simulink model "STEVE_ver28"  (R2022a)
settings: Solver=VariableStepAuto  StartTime=0.0  StopTime=Stop_Time  FixedStep=0.000001  RelTol=1e-5
values from neighbouring files (symbols this model uses):
  Bed_ave_OD = (1+Bed_ins_OD)/2    (= 1.667)    [STEVE_initialization.m]    (also in STEVE_running.m = (1+Bed_ins_OD)/2; STEVE_v4_C1Demo_2023_Nominal.m)
  Bed_ins_OD = 2.334    [STEVE_initialization.m]    (also in STEVE_v4_C1Demo_2023_Nominal.m)
  Bed_thickness = 0.049    [STEVE_initialization.m]    (also in STEVE_v4_C1Demo_2023_Nominal.m)
  Belimo_Cv = 16    [STEVE_initialization.m]    (also in STEVE_v4_C1Demo_2023_Nominal.m)
  flow_rate = 8    [STEVE_initialization.m]    (also in STEVE_v4_C1Demo_2023_Nominal.m)
  Heat_ads = 40000    [STEVE_initialization.m]    (also in STEVE_v4_C1Demo_2023_Nominal.m)
  Heater_output = 85.3    [STEVE_initialization.m]    (also in STEVE_v4_C1Demo_2023_Nominal.m)
  L = 0.508    [STEVE_initialization.m]    (also in STEVE_v4_C1Demo_2023_Nominal.m)
  L_inch = L*39.3701    (= 20.0000108)    [STEVE_initialization.m]    (also in STEVE_v4_C1Demo_2023_Nominal.m)
  max_temp = 200+273.15    (= 473.15)    [STEVE_initialization.m]    (also in STEVE_v4_C1Demo_2023_Nominal.m)
  mesh_size = 15    [STEVE_initialization.m]    (also in STEVE_v4_C1Demo_2023_Nominal.m)
  Pipe_ave_HD = (pipe_HD+0.5)/2    (= 0.465)    [STEVE_initialization.m]    (also in STEVE_running.m = (pipe_HD+0.5)/2; STEVE_v4_C1Demo_2023_Nominal.m)
  pipe_HD = 0.43    [STEVE_initialization.m]    (also in STEVE_v4_C1Demo_2023_Nominal.m)
  Ramp_rate = 0.0833    [STEVE_initialization.m]    (also in STEVE_v4_C1Demo_2023_Nominal.m)
  room_pressure = 13.3    [STEVE_initialization.m]    (also in STEVE_v4_C1Demo_2023_Nominal.m)
  t_Total = Adsorption_time + FlowStop_time + Valve_close_Time + Select_valve_close_Time + Pump_down_time + Desorption_time + SelectValve_open_Time + Valve_open_Time    (= 9635)    [STEVE_initialization.m]    (also in STEVE_running.m = Adsorption_time + FlowStop_time + Valve_close_Time + Select_; STEVE_v4_C1Demo_2023_Nominal.m)
libraries: fl_lib x229, nesl_utility x75, slpidlib x2
(part 4 of 5)

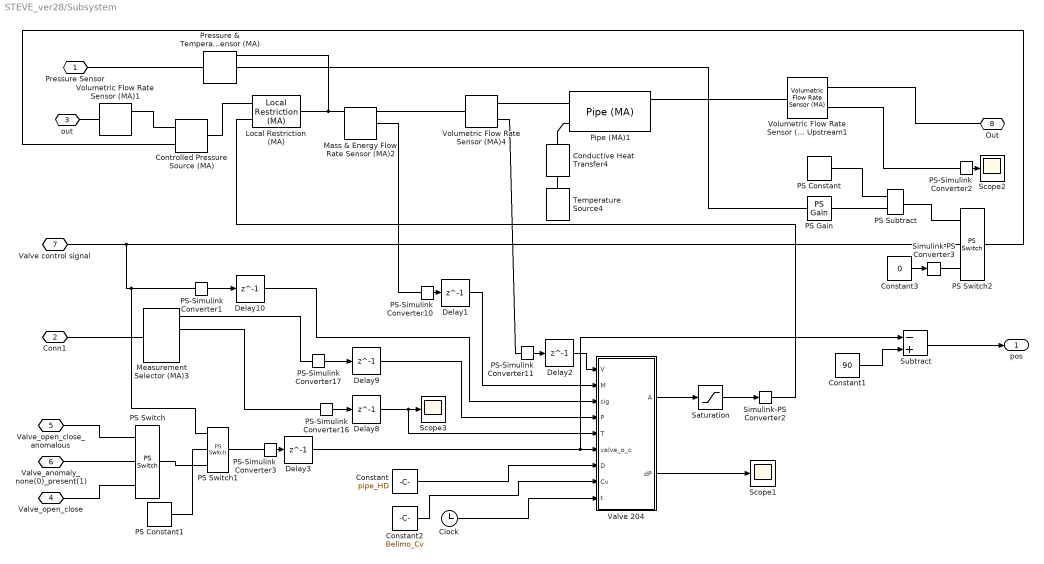
== system STEVE_ver28/Subsystem ==
  Clock : Clock
  Conductive Heat Transfer4 : fl_lib/Thermal/Thermal Elements/Conductive Heat Transfer  area=51.8 in^2  thickness=pipe_wall in  th_cond=pipe_tc W/(m*K)  T_specify=off  T_priority=None  T=0 K  T_nominal_specify=off  T_nominal_unit=K  T_nominal_value=1  Q_specify=off  Q_priority=None  Q=0 W  Q_nominal_specify=off  Q_nominal_unit=W  Q_nominal_value=1
      settings: SourceProductBaseCode=PW,SS,VE
  Constant : Constant  Value=pipe_HD
  Constant1 : Constant  Value=90
  Constant2 : Constant  Value=Belimo_Cv
  Constant3 : Constant  Value=0
  Controlled Pressure Source (MA) : fl_lib/Moist Air/Sources/Controlled Pressure Source (MA)  power_spec=foundation.enum.power_spec.isentropic  area_A=(pi*pipe_HD^2)/4 in^2  area_B=(pi*pipe_HD^2)/4 in^2
      settings: SourceProductBaseCode=PW,SS,VE  InternalSimscapePortConfiguration="{\"Bottom\":[],\"Left\":[{\"id\":\"A\",\"label\":\"A\",\"type\":\"foundation.moist_air.moist_air\"},{\"id\":\"P\",\"label\":\"P\",\"type\":\"input\"}],\"Right\":[{\"id\":\"B\",\"label\":\"B\",\"type\":\"foundation.moist_air.moist_air\"}],\"Top\":[]}"
  Delay1 : Delay  DelayLength=1  InitialCondition=0
  Delay10 : Delay  DelayLength=1  InitialCondition=0
  Delay2 : Delay  DelayLength=1  InitialCondition=0.00013
  Delay3 : Delay  DelayLength=1  InitialCondition=18
  Delay8 : Delay  DelayLength=1  InitialCondition=293
  Delay9 : Delay  DelayLength=1  InitialCondition=90000
  Local Restriction (MA) : fl_lib/Moist Air/Elements/Local Restriction (MA)  restriction_type=foundation.enum.restriction_type.variable  restriction_area=0.001 m^2  min_area=1e-20 in^2  max_area=(pi*(pipe_HD-0.0001)^2)/4 in^2  area=(pi*pipe_HD^2)/4 in^2  Cd=0.64  B_lam=0.999
      settings: SourceProductBaseCode=PW,SS,VE
  Mass & Energy Flow Rate Sensor (MA)2 : fl_lib/Moist Air/Sensors/Mass & Energy Flow Rate Sensor (MA)
      settings: SourceProductBaseCode=PW,SS,VE  InternalSimscapePortConfiguration="{\"Bottom\":[],\"Left\":[{\"id\":\"A\",\"label\":\"A\",\"type\":\"foundation.moist_air.moist_air\"},{\"id\":\"Mw\",\"label\":\"Mw\",\"type\":\"output\"},{\"id\":\"Mg\",\"label\":\"Mg\",\"type\":\"output\"}],\"Right\":[{\"id\":\"B\",\"label\":\"B\",\"type\":\"foundation.moist_air.moist_air\"},{\"id\":\"M\",\"label\":\"M\",\"type\":\"output\"},{\"id\":\"PHI\",\"label\":\"Phi\",\"type\":\"output\"}],\"Top\":[]}"
  Measurement Selector (MA)3 : fl_lib/Moist Air/Sensors/Measurement Selector (MA)  moisture_spec=foundation.enum.moisture_spec.relative_humidity  trace_gas_spec=foundation.enum.trace_gas_spec.mole_fraction
      settings: SourceProductBaseCode=PW,SS,VE
  PS Constant : fl_lib/Physical Signals/Sources/PS Constant  constant=0 Pa
      settings: SourceProductBaseCode=PW,SS,VE
  PS Constant1 : fl_lib/Physical Signals/Sources/PS Constant  constant=0
      settings: SourceProductBaseCode=PW,SS,VE
  PS Gain : fl_lib/Physical Signals/Functions/PS Gain  gain=1
      settings: SourceProductBaseCode=PW,SS,VE
  PS Subtract : fl_lib/Physical Signals/Functions/PS Subtract
      settings: SourceProductBaseCode=PW,SS,VE
  PS Switch : fl_lib/Physical Signals/Nonlinear Operators/PS Switch  Threshold=1
      settings: SourceProductBaseCode=PW,SS,VE  InternalSimscapePortConfiguration="{\"Bottom\":[],\"Left\":[{\"id\":\"I1\",\"label\":\"\",\"type\":\"input\"},{\"id\":\"I2\",\"label\":\"\",\"type\":\"input\"},{\"id\":\"I3\",\"label\":\"\",\"type\":\"input\"}],\"Right\":[{\"id\":\"O\",\"label\":\"\",\"type\":\"output\"}],\"Top\":[]}"
  PS Switch1 : fl_lib/Physical Signals/Nonlinear Operators/PS Switch  Threshold=1
      settings: SourceProductBaseCode=PW,SS,VE  InternalSimscapePortConfiguration="{\"Bottom\":[],\"Left\":[{\"id\":\"I1\",\"label\":\"\",\"type\":\"input\"},{\"id\":\"I2\",\"label\":\"\",\"type\":\"input\"},{\"id\":\"I3\",\"label\":\"\",\"type\":\"input\"}],\"Right\":[{\"id\":\"O\",\"label\":\"\",\"type\":\"output\"}],\"Top\":[]}"
  PS Switch2 : fl_lib/Physical Signals/Nonlinear Operators/PS Switch  Threshold=1
      settings: SourceProductBaseCode=PW,SS,VE  InternalSimscapePortConfiguration="{\"Bottom\":[],\"Left\":[{\"id\":\"I1\",\"label\":\"\",\"type\":\"input\"},{\"id\":\"I2\",\"label\":\"\",\"type\":\"input\"},{\"id\":\"I3\",\"label\":\"\",\"type\":\"input\"}],\"Right\":[{\"id\":\"O\",\"label\":\"\",\"type\":\"output\"}],\"Top\":[]}"
  PS-Simulink Converter{1,3,10..11,16..17} (6 alike) : nesl_utility/PS-Simulink Converter  PhysicalDomain=network_engine_domain  SubClassName=ps_output  LeftPortType=input  RightPortType=output  PseudoPeriodic=off  Frequencies=[]  VectorFormat=1-D array  Unit=inherit  AffineConversion=off
      settings: SourceProductBaseCode=SS,PW,VE
  PS-Simulink Converter2 : nesl_utility/PS-Simulink Converter  PhysicalDomain=network_engine_domain  SubClassName=ps_output  LeftPortType=input  RightPortType=output  PseudoPeriodic=off  Frequencies=[]  VectorFormat=1-D array  Unit=lpm  AffineConversion=off
      settings: SourceProductBaseCode=SS,PW,VE
  Pipe (MA)1 : fl_lib/Moist Air/Elements/Pipe (MA)  length=16.5 in  area=(pi*pipe_HD^2)/4 in^2  Dh=pipe_HD in  length_add=0.1 m  roughness=roughness m  Re_lam=2000  Re_tur=4000  shape_factor=64  Nu_lam=3.66  RH_ws=1  time_constant=1e-3 s  moisture_trace_gas_source=foundation.enum.moisture_trace_gas_source.none  moisture_source_spec=foundation.enum.moisture_source_spec.vapor  moisture_mass_flow=0 kg/s  moisture_temperature_spec=foundation.enum.temperature_spec.atmospheric  moisture_temperature=293.15 K  trace_gas_mass_flow=0 kg/s  trace_gas_temperature_spec=foundation.enum.temperature_spec.atmospheric  trace_gas_temperature=293.15 K  p_I_specify=off  p_I_priority=High  p_I=0.101325 MPa  p_I_nominal_specify=off  p_I_nominal_unit=MPa  p_I_nominal_value=1  T_I_specify=off  T_I_priority=High  T_I=293.15 K  T_I_nominal_specify=off  T_I_nominal_unit=K  T_I_nominal_value=1  RH_I_specify=off  RH_I_priority=High  RH_I=0  RH_I_nominal_specify=off  RH_I_nominal_unit=1  RH_I_nominal_value=1  x_w_I_specify=off  x_w_I_priority=None  x_w_I=0  x_w_I_nominal_specify=off  x_w_I_nominal_unit=1  x_w_I_nominal_value=1  y_w_I_specify=off  y_w_I_priority=None  y_w_I=0  y_w_I_nominal_specify=off  y_w_I_nominal_unit=1  y_w_I_nominal_value=1  HR_I_specify=off  HR_I_priority=None  HR_I=0  HR_I_nominal_specify=off  HR_I_nominal_unit=1  HR_I_nominal_value=1  x_g_I_specify=off  x_g_I_priority=High  x_g_I=0  x_g_I_nominal_specify=off  x_g_I_nominal_unit=1  x_g_I_nominal_value=1  y_g_I_specify=off  y_g_I_priority=None  y_g_I=0  y_g_I_nominal_specify=off  y_g_I_nominal_unit=1  y_g_I_nominal_value=1
      settings: SourceProductBaseCode=PW,SS,VE
  Pressure & Temperature Sensor (MA) : fl_lib/Moist Air/Sensors/Pressure & Temperature Sensor (MA)
      settings: SourceProductBaseCode=PW,SS,VE  InternalSimscapePortConfiguration="{\"Bottom\":[],\"Left\":[{\"id\":\"A\",\"label\":\"A\",\"type\":\"foundation.moist_air.moist_air\"}],\"Right\":[{\"id\":\"B\",\"label\":\"B\",\"type\":\"foundation.moist_air.moist_air\"},{\"id\":\"P\",\"label\":\"P\",\"type\":\"output\"},{\"id\":\"T\",\"label\":\"T\",\"type\":\"output\"}],\"Top\":[]}"
  Saturation : Saturate  UpperLimit=inf  LowerLimit=1e-10
  Scope1 : Scope
  Scope2 : Scope
  Scope3 : Scope
  Simulink-PS Converter2 : nesl_utility/Simulink-PS Converter  PhysicalDomain=network_engine_domain  SubClassName=ps_input  LeftPortType=input  RightPortType=output  PseudoPeriodic=off  Frequencies=[]  NoiseDistribution=none  NoiseParameters=[]  Unit=1  AffineConversion=off  FilteringAndDerivatives=provide  SimscapeFilterOrder=1  InputFilterTimeConstant=0.001  UdotUserProvided=0
      settings: SourceProductBaseCode=SS,PW,VE
  Simulink-PS Converter3 : nesl_utility/Simulink-PS Converter  PhysicalDomain=network_engine_domain  SubClassName=ps_input  LeftPortType=input  RightPortType=output  PseudoPeriodic=off  Frequencies=[]  NoiseDistribution=none  NoiseParameters=[]  Unit=Pa  AffineConversion=off  FilteringAndDerivatives=provide  SimscapeFilterOrder=1  InputFilterTimeConstant=0.001  UdotUserProvided=0
      settings: SourceProductBaseCode=SS,PW,VE
  Subtract : Sum  Inputs=-+
  Temperature Source4 : fl_lib/Thermal/Thermal Sources/Temperature Source  temperature=room_temp K
      settings: SourceProductBaseCode=PW,SS,VE
  Valve 204 : MATLAB Function  TreatAsAtomicUnit=on
  Volumetric Flow Rate Sensor (MA) Upstream1 : fl_lib/Moist Air/Sensors/Volumetric Flow Rate Sensor (MA)  volumetric_flow_conditions=foundation.enum.volumetric_flow_conditions.actual  p_std=0.101325 MPa  T_std=20 degC  RH_std=0.65
      settings: SourceProductBaseCode=PW,SS,VE  InternalSimscapePortConfiguration="{\"Bottom\":[],\"Left\":[{\"id\":\"A\",\"label\":\"A\",\"type\":\"foundation.moist_air.moist_air\"}],\"Right\":[{\"id\":\"B\",\"label\":\"B\",\"type\":\"foundation.moist_air.moist_air\"},{\"id\":\"V\",\"label\":\"V\",\"type\":\"output\"}],\"Top\":[]}"
  Volumetric Flow Rate Sensor (MA)1 : fl_lib/Moist Air/Sensors/Volumetric Flow Rate Sensor (MA)  volumetric_flow_conditions=foundation.enum.volumetric_flow_conditions.actual  p_std=0.101325 MPa  T_std=20 degC  RH_std=0.65
      settings: SourceProductBaseCode=PW,SS,VE  InternalSimscapePortConfiguration="{\"Bottom\":[],\"Left\":[{\"id\":\"A\",\"label\":\"A\",\"type\":\"foundation.moist_air.moist_air\"}],\"Right\":[{\"id\":\"B\",\"label\":\"B\",\"type\":\"foundation.moist_air.moist_air\"},{\"id\":\"V\",\"label\":\"V\",\"type\":\"output\"}],\"Top\":[]}"
  Volumetric Flow Rate Sensor (MA)4 : fl_lib/Moist Air/Sensors/Volumetric Flow Rate Sensor (MA)  volumetric_flow_conditions=foundation.enum.volumetric_flow_conditions.actual  p_std=0.101325 MPa  T_std=20 degC  RH_std=0.65
      settings: SourceProductBaseCode=PW,SS,VE  InternalSimscapePortConfiguration="{\"Bottom\":[],\"Left\":[{\"id\":\"A\",\"label\":\"A\",\"type\":\"foundation.moist_air.moist_air\"}],\"Right\":[{\"id\":\"B\",\"label\":\"B\",\"type\":\"foundation.moist_air.moist_air\"},{\"id\":\"V\",\"label\":\"V\",\"type\":\"output\"}],\"Top\":[]}"
  Pressure Sensor : PMIOPort  Side=Left
  Conn1 : PMIOPort  Port=2  Side=Left
  out : PMIOPort  Port=3  Side=Left
  Valve_open_close : PMIOPort  Port=4  Side=Left
  Valve_open_close_anomalous : PMIOPort  Port=5  Side=Left
  Valve_anomaly_none(0)_present(1) : PMIOPort  Port=6  Side=Left
  Valve control signal : PMIOPort  Port=7  Side=Left
  Out : PMIOPort  Port=8  Side=Right
  pos : Outport
  wires:
  PS-Simulink Converter2/1 -> Scope2/1
  Constant/1 -> Valve 204/7(D)
  PS-Simulink Converter3/1 -> Delay3/1
  PS-Simulink Converter10/1 -> Delay1/1
  PS-Simulink Converter11/1 -> Delay2/1
  Delay1/1 -> Valve 204/2(M)
  Delay2/1 -> Valve 204/1(V)
  PS-Simulink Converter16/1 -> Delay8/1
  Delay8/1 -> Valve 204/5(T), Scope3/1
  Constant2/1 -> Valve 204/8(Cv)
  PS-Simulink Converter17/1 -> Delay9/1
  Delay9/1 -> Valve 204/4(P)
  PS-Simulink Converter1/1 -> Delay10/1
  Delay10/1 -> Valve 204/3(sig)
  Valve 204/2(dP) -> Scope1/1
  Clock/1 -> Valve 204/9(t)
  Constant3/1 -> Simulink-PS Converter3/1
  Saturation/1 -> Simulink-PS Converter2/1
  Valve 204/1(A) -> Saturation/1
  Delay3/1 -> Subtract/1, Valve 204/6(valve_o_c)
  Subtract/1 -> pos/1
  Constant1/1 -> Subtract/2
  connections:
  Conductive Heat Transfer4/LConn1 -- Pipe (MA)1/LConn2
  Temperature Source4/LConn1 -- Conductive Heat Transfer4/RConn1
  Volumetric Flow Rate Sensor (MA) Upstream1/RConn1 -- Out/RConn1
  PS-Simulink Converter2/LConn1 -- Volumetric Flow Rate Sensor (MA) Upstream1/RConn2
  Volumetric Flow Rate Sensor (MA)1/LConn1 -- out/RConn1
  Valve_anomaly_none(0)_present(1)/RConn1 -- PS Switch/LConn2
  Simulink-PS Converter2/RConn1 -- Local Restriction (MA)/LConn2
  Valve_open_close_anomalous/RConn1 -- PS Switch/LConn1
  Valve_open_close/RConn1 -- PS Switch/LConn3
  Mass & Energy Flow Rate Sensor (MA)2/RConn1 -- Volumetric Flow Rate Sensor (MA)4/LConn1
  Volumetric Flow Rate Sensor (MA)4/RConn1 -- Pipe (MA)1/LConn1
  Mass & Energy Flow Rate Sensor (MA)2/RConn2 -- PS-Simulink Converter10/LConn1
  Volumetric Flow Rate Sensor (MA)4/RConn2 -- PS-Simulink Converter11/LConn1
  Measurement Selector (MA)3/RConn2 -- PS-Simulink Converter16/LConn1
  Measurement Selector (MA)3/RConn1 -- PS-Simulink Converter17/LConn1
  PS-Simulink Converter1/LConn1 -- PS Switch1/LConn1 -- PS Switch2/LConn2 -- Valve control signal/RConn1
  Mass & Energy Flow Rate Sensor (MA)2/LConn1 -- Pressure & Temperature Sensor (MA)/RConn1 -- Local Restriction (MA)/RConn1
  PS Switch2/RConn1 -- Controlled Pressure Source (MA)/LConn2
  Simulink-PS Converter3/RConn1 -- PS Switch2/LConn3
  Volumetric Flow Rate Sensor (MA) Upstream1/LConn1 -- Pipe (MA)1/RConn1
  Controlled Pressure Source (MA)/LConn1 -- Volumetric Flow Rate Sensor (MA)1/RConn1
  Controlled Pressure Source (MA)/RConn1 -- Local Restriction (MA)/LConn1
  Pressure & Temperature Sensor (MA)/RConn2 -- PS Gain/LConn1
  PS Subtract/RConn1 -- PS Switch2/LConn1
  PS Subtract/LConn1 -- PS Constant/RConn1
  PS Gain/RConn1 -- PS Subtract/LConn2
  Pressure Sensor/RConn1 -- Pressure & Temperature Sensor (MA)/LConn1
  Conn1/RConn1 -- Measurement Selector (MA)3/LConn1
  PS Switch1/RConn1 -- PS-Simulink Converter3/LConn1
  PS Constant1/RConn1 -- PS Switch1/LConn2
  PS Switch1/LConn3 -- PS Switch/RConn1

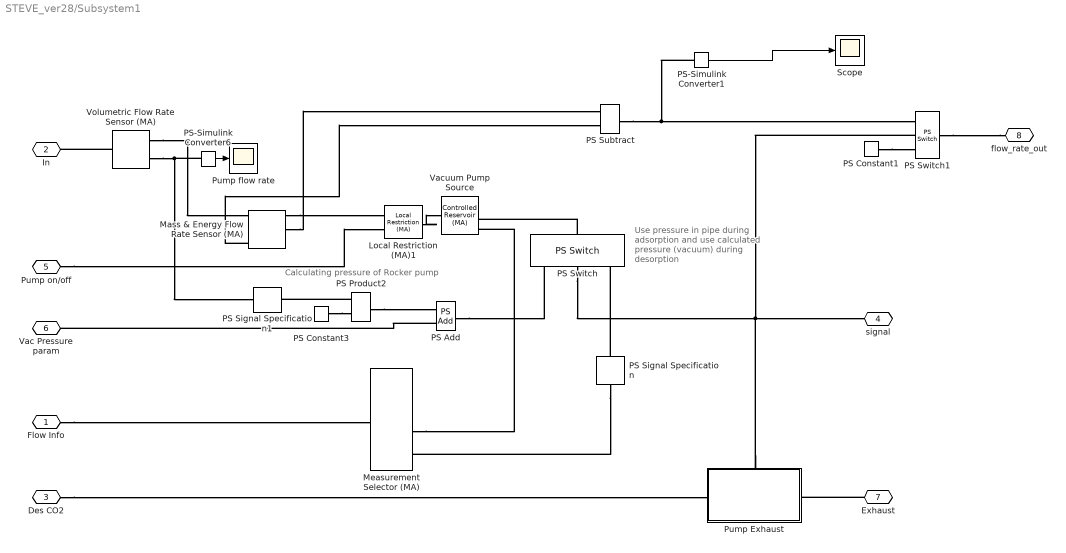
== system STEVE_ver28/Subsystem1 ==
  note: Use pressure in pipe during adsorption and use calculated pressure (vacuum) during desorption
  note: Calculating pressure of Rocker pump
  Local Restriction (MA)1 : fl_lib/Moist Air/Elements/Local Restriction (MA)  restriction_type=foundation.enum.restriction_type.variable  restriction_area=0.001 m^2  min_area=1e-10 in^2  max_area=(pi*(pipe_HD-0.0001)^2)/4 in^2  area=(pi*pipe_HD^2)/4 in^2  Cd=0.64  B_lam=0.999
      settings: SourceProductBaseCode=PW,SS,VE
  Mass & Energy Flow Rate Sensor (MA) : fl_lib/Moist Air/Sensors/Mass & Energy Flow Rate Sensor (MA)
      settings: SourceProductBaseCode=PW,SS,VE  InternalSimscapePortConfiguration="{\"Bottom\":[],\"Left\":[{\"id\":\"A\",\"label\":\"A\",\"type\":\"foundation.moist_air.moist_air\"},{\"id\":\"Mw\",\"label\":\"Mw\",\"type\":\"output\"},{\"id\":\"Mg\",\"label\":\"Mg\",\"type\":\"output\"}],\"Right\":[{\"id\":\"B\",\"label\":\"B\",\"type\":\"foundation.moist_air.moist_air\"},{\"id\":\"M\",\"label\":\"M\",\"type\":\"output\"},{\"id\":\"PHI\",\"label\":\"Phi\",\"type\":\"output\"}],\"Top\":[]}"
  Measurement Selector (MA) : fl_lib/Moist Air/Sensors/Measurement Selector (MA)  moisture_spec=foundation.enum.moisture_spec.relative_humidity  trace_gas_spec=foundation.enum.trace_gas_spec.mole_fraction
      settings: SourceProductBaseCode=PW,SS,VE
  PS Add : fl_lib/Physical Signals/Functions/PS Add
      settings: SourceProductBaseCode=PW,SS,VE
  PS Constant1 : fl_lib/Physical Signals/Sources/PS Constant  constant=0 kg/s
      settings: SourceProductBaseCode=PW,SS,VE
  PS Constant3 : fl_lib/Physical Signals/Sources/PS Constant  constant=60000*2055.44
      settings: SourceProductBaseCode=PW,SS,VE
  PS Product2 : fl_lib/Physical Signals/Functions/PS Product
      settings: SourceProductBaseCode=PW,SS,VE
  PS Signal Specification : fl_lib/Physical Signals/Utilities/PS Signal Specification  signalType=zeros(1, 1)
      settings: SourceProductBaseCode=PW,SS,VE  InternalSimscapePortConfiguration="{\"Bottom\":[],\"Left\":[{\"id\":\"I\",\"label\":\"\",\"type\":\"input\"}],\"Right\":[{\"id\":\"O\",\"label\":\"\",\"type\":\"output\"}],\"Top\":[]}"
  PS Signal Specification1 : fl_lib/Physical Signals/Utilities/PS Signal Specification  signalType=zeros(1, 1)
      settings: SourceProductBaseCode=PW,SS,VE  InternalSimscapePortConfiguration="{\"Bottom\":[],\"Left\":[{\"id\":\"I\",\"label\":\"\",\"type\":\"input\"}],\"Right\":[{\"id\":\"O\",\"label\":\"\",\"type\":\"output\"}],\"Top\":[]}"
  PS Subtract : fl_lib/Physical Signals/Functions/PS Subtract
      settings: SourceProductBaseCode=PW,SS,VE
  PS Switch : fl_lib/Physical Signals/Nonlinear Operators/PS Switch  Threshold=1
      settings: SourceProductBaseCode=PW,SS,VE  InternalSimscapePortConfiguration="{\"Bottom\":[],\"Left\":[{\"id\":\"I1\",\"label\":\"\",\"type\":\"input\"},{\"id\":\"I2\",\"label\":\"\",\"type\":\"input\"},{\"id\":\"I3\",\"label\":\"\",\"type\":\"input\"}],\"Right\":[{\"id\":\"O\",\"label\":\"\",\"type\":\"output\"}],\"Top\":[]}"
  PS Switch1 : fl_lib/Physical Signals/Nonlinear Operators/PS Switch  Threshold=1
      settings: SourceProductBaseCode=PW,SS,VE  InternalSimscapePortConfiguration="{\"Bottom\":[],\"Left\":[{\"id\":\"I1\",\"label\":\"\",\"type\":\"input\"},{\"id\":\"I2\",\"label\":\"\",\"type\":\"input\"},{\"id\":\"I3\",\"label\":\"\",\"type\":\"input\"}],\"Right\":[{\"id\":\"O\",\"label\":\"\",\"type\":\"output\"}],\"Top\":[]}"
  PS-Simulink Converter1 : nesl_utility/PS-Simulink Converter  PhysicalDomain=network_engine_domain  SubClassName=ps_output  LeftPortType=input  RightPortType=output  PseudoPeriodic=off  Frequencies=[]  VectorFormat=1-D array  Unit=inherit  AffineConversion=off
      settings: SourceProductBaseCode=SS,PW,VE
  PS-Simulink Converter6 : nesl_utility/PS-Simulink Converter  PhysicalDomain=network_engine_domain  SubClassName=ps_output  LeftPortType=input  RightPortType=output  PseudoPeriodic=off  Frequencies=[]  VectorFormat=1-D array  Unit=inherit  AffineConversion=off
      settings: SourceProductBaseCode=SS,PW,VE
  Pump Exhaust : Subsystem
      settings: PortSchema="{\"entries\":[{\"content\":{\"sides\":[{\"content\":{\"connectorIds\":[\"LConn1\"]},\"type\":\"ConnectorPlacement.EquallySpacedRectSide\",\"uuid\":\"b2354edd-b543-4edf-a01b-db30485ad618\"},{\"content\":{\"connectorIds\":[\"RConn1\"],\"side\":\"RIGHT\"},\"type\":\"ConnectorPlacement.EquallySpacedRectSide\",\"uuid\":\"d9a43c3a-66fb-4531-b80b-3879ed72e7c6\"},{\"content\":{\"connectorIds\":[\"LConn2\"],\"side\":\"TOP\"},\"type\":\"ConnectorPlacement.EquallySpacedRectSide\",\"uuid\":\"dc87ddbc-b19b-4cef-a55e-d823cd2e963a\"}]},\"type\":\"ConnectorPlacement.EquallySpacedConnector\",\"uuid\":\"b555a200-7821-430f-8e9a-b812e79bdcb3\"}],\"packageUris\":[\"http://schema.mathworks.com/mf0/Connector/R2020b\"],\"version\":\"1.0\"}"
  Pump flow rate : Scope
  Scope : Scope
  Vacuum Pump Source : fl_lib/Moist Air/Elements/Controlled Reservoir (MA)  moisture_spec=foundation.enum.moisture_spec.relative_humidity  trace_gas_spec=foundation.enum.trace_gas_spec.mole_fraction  RH_ws=1  area_A=(pi*pipe_HD^2)/4 in^2  input_error_spec=foundation.enum.input_range_error.warn
      settings: SourceProductBaseCode=PW,SS,VE  InternalSimscapePortConfiguration="{\"Bottom\":[],\"Left\":[{\"id\":\"A\",\"label\":\"A\",\"type\":\"foundation.moist_air.moist_air\"}],\"Right\":[{\"id\":\"T\",\"label\":\"T\",\"type\":\"input\"},{\"id\":\"P\",\"label\":\"P\",\"type\":\"input\"},{\"id\":\"W\",\"label\":\"W\",\"type\":\"input\"},{\"id\":\"G\",\"label\":\"G\",\"type\":\"input\"}],\"Top\":[]}"
  Volumetric Flow Rate Sensor (MA) : fl_lib/Moist Air/Sensors/Volumetric Flow Rate Sensor (MA)  volumetric_flow_conditions=foundation.enum.volumetric_flow_conditions.actual  p_std=0.101325 MPa  T_std=20 degC  RH_std=0.65
      settings: SourceProductBaseCode=PW,SS,VE  InternalSimscapePortConfiguration="{\"Bottom\":[],\"Left\":[{\"id\":\"A\",\"label\":\"A\",\"type\":\"foundation.moist_air.moist_air\"}],\"Right\":[{\"id\":\"B\",\"label\":\"B\",\"type\":\"foundation.moist_air.moist_air\"},{\"id\":\"V\",\"label\":\"V\",\"type\":\"output\"}],\"Top\":[]}"
  Flow Info : PMIOPort  Side=Left
  In : PMIOPort  Port=2  Side=Left
  Des CO2 : PMIOPort  Port=3  Side=Left
  signal : PMIOPort  Port=4  Side=Right
  Pump on/off : PMIOPort  Port=5  Side=Right
  Vac Pressure param : PMIOPort  Port=6  Side=Right
  Exhaust : PMIOPort  Port=7  Side=Right
  flow_rate_out : PMIOPort  Port=8  Side=Right
  wires:
  PS-Simulink Converter6/1 -> Pump flow rate/1
  PS-Simulink Converter1/1 -> Scope/1
  connections:
  Flow Info/RConn1 -- Measurement Selector (MA)/LConn1
  PS Signal Specification/LConn1 -- Measurement Selector (MA)/RConn1
  Measurement Selector (MA)/RConn2 -- Vacuum Pump Source/RConn1
  PS Switch/LConn2 -- PS Switch1/LConn2 -- Pump Exhaust/LConn2 -- signal/RConn1
  PS Switch/RConn1 -- Vacuum Pump Source/RConn2
  PS Signal Specification/RConn1 -- PS Switch/LConn3
  Pump on/off/RConn1 -- Local Restriction (MA)1/LConn2
  Volumetric Flow Rate Sensor (MA)/LConn1 -- In/RConn1
  PS Product2/LConn1 -- PS Signal Specification1/RConn1
  Volumetric Flow Rate Sensor (MA)/RConn2 -- PS-Simulink Converter6/LConn1 -- PS Signal Specification1/LConn1
  Des CO2/RConn1 -- Pump Exhaust/LConn1
  Exhaust/RConn1 -- Pump Exhaust/RConn1
  Local Restriction (MA)1/RConn1 -- Vacuum Pump Source/LConn1
  Mass & Energy Flow Rate Sensor (MA)/RConn1 -- Local Restriction (MA)1/LConn1
  Volumetric Flow Rate Sensor (MA)/RConn1 -- Mass & Energy Flow Rate Sensor (MA)/LConn1
  Mass & Energy Flow Rate Sensor (MA)/RConn2 -- PS Subtract/LConn1
  PS Constant1/RConn1 -- PS Switch1/LConn3
  PS Subtract/RConn1 -- PS-Simulink Converter1/LConn1 -- PS Switch1/LConn1
  PS Switch1/RConn1 -- flow_rate_out/RConn1
  Mass & Energy Flow Rate Sensor (MA)/LConn3 -- PS Subtract/LConn2
  PS Add/RConn1 -- PS Switch/LConn1
  PS Constant3/RConn1 -- PS Product2/LConn2
  PS Add/LConn2 -- Vac Pressure param/RConn1
  PS Product2/RConn1 -- PS Add/LConn1

== system STEVE_ver28/Upstream Sensors ==
  note: Measurement
      | Selector Block
  Measurement Selector (MA) : fl_lib/Moist Air/Sensors/Measurement Selector (MA)  moisture_spec=foundation.enum.moisture_spec.relative_humidity  trace_gas_spec=foundation.enum.trace_gas_spec.mole_fraction
      settings: SourceProductBaseCode=PW,SS,VE
  PS-Simulink Converter2 : nesl_utility/PS-Simulink Converter  PhysicalDomain=network_engine_domain  SubClassName=ps_output  LeftPortType=input  RightPortType=output  PseudoPeriodic=off  Frequencies=[]  VectorFormat=1-D array  Unit=lpm  AffineConversion=off
      settings: SourceProductBaseCode=SS,PW,VE
  Scope2 : Scope
  Volumetric Flow Rate Sensor (MA) Upstream2 : fl_lib/Moist Air/Sensors/Volumetric Flow Rate Sensor (MA)  volumetric_flow_conditions=foundation.enum.volumetric_flow_conditions.actual  p_std=0.101325 MPa  T_std=20 degC  RH_std=0.65
      settings: SourceProductBaseCode=PW,SS,VE  InternalSimscapePortConfiguration="{\"Bottom\":[],\"Left\":[{\"id\":\"A\",\"label\":\"A\",\"type\":\"foundation.moist_air.moist_air\"}],\"Right\":[{\"id\":\"B\",\"label\":\"B\",\"type\":\"foundation.moist_air.moist_air\"},{\"id\":\"V\",\"label\":\"V\",\"type\":\"output\"}],\"Top\":[]}"
  In : PMIOPort  Side=Left
  Sensor In : PMIOPort  Port=2  Side=Left
  Out : PMIOPort  Port=3  Side=Right
  CO2_out : PMIOPort  Port=4  Side=Right
  Upstream Pressure : PMIOPort  Port=5  Side=Right
  RH Out : PMIOPort  Port=6  Side=Right
  Upstream Temperature : PMIOPort  Port=7  Side=Right
  wires:
  PS-Simulink Converter2/1 -> Scope2/1
  connections:
  Measurement Selector (MA)/RConn3 -- RH Out/RConn1
  Out/RConn1 -- Volumetric Flow Rate Sensor (MA) Upstream2/RConn1
  In/RConn1 -- Volumetric Flow Rate Sensor (MA) Upstream2/LConn1
  PS-Simulink Converter2/LConn1 -- Volumetric Flow Rate Sensor (MA) Upstream2/RConn2
  Measurement Selector (MA)/RConn1 -- Upstream Pressure/RConn1
  Measurement Selector (MA)/LConn1 -- Sensor In/RConn1
  Upstream Temperature/RConn1 -- Measurement Selector (MA)/RConn2
  Measurement Selector (MA)/RConn4 -- CO2_out/RConn1

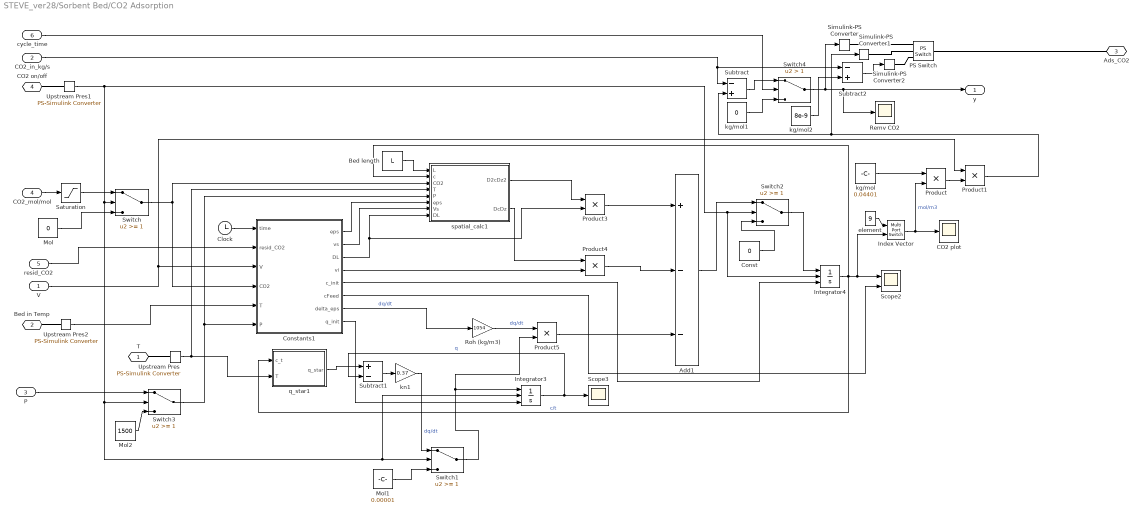
== system STEVE_ver28/Sorbent Bed/CO2 Adsorption ==
  V : Inport
  CO2_in_kg/s : Inport  Port=2
  P : Inport  Port=3
  CO2_mol/mol : Inport  Port=4
  resid_CO2 : Inport  Port=5
  cycle_time : Inport  Port=6
  Add1 : Sum  Inputs=+--
  Bed length : Constant  Value=L
  CO2 plot : Scope
  Clock : Clock
  Const : Constant  Value=0
  Constants1 : MATLAB Function  TreatAsAtomicUnit=on
  Index Vector : MultiPortSwitch  Inputs=1  SaturateOnIntegerOverflow=off  InputSameDT=off
  Integrator3 : Integrator  ExternalReset=either  InitialConditionSource=external  InitialCondition=zeros(10,1)
  Integrator4 : Integrator  ExternalReset=either  InitialConditionSource=external  InitialCondition=0.003
  Mol : Constant  Value=0
  Mol1 : Constant  Value=0.00001
  Mol2 : Constant  Value=1500
  PS Switch : fl_lib/Physical Signals/Nonlinear Operators/PS Switch  Threshold=8e-9 kg/s
      settings: SourceProductBaseCode=PW,SS,VE  InternalSimscapePortConfiguration="{\"Bottom\":[],\"Left\":[{\"id\":\"I1\",\"label\":\"\",\"type\":\"input\"},{\"id\":\"I2\",\"label\":\"\",\"type\":\"input\"},{\"id\":\"I3\",\"label\":\"\",\"type\":\"input\"}],\"Right\":[{\"id\":\"O\",\"label\":\"\",\"type\":\"output\"}],\"Top\":[]}"
  Product{,1,3..5} (5 alike) : Product
  Remv CO2 : Scope
  Roh (kg/m3) : Gain  Gain=1054
  Saturation : Saturate  UpperLimit=0.003  LowerLimit=-inf
  Scope2 : Scope  NumInputPorts=2
  Scope3 : Scope
  Simulink-PS Converter : nesl_utility/Simulink-PS Converter  PhysicalDomain=network_engine_domain  SubClassName=ps_input  LeftPortType=input  RightPortType=output  PseudoPeriodic=off  Frequencies=[]  NoiseDistribution=none  NoiseParameters=[]  Unit=kg/s  AffineConversion=off  FilteringAndDerivatives=provide  SimscapeFilterOrder=1  InputFilterTimeConstant=0.001  UdotUserProvided=0
      settings: SourceProductBaseCode=SS,PW,VE
  Simulink-PS Converter1 : nesl_utility/Simulink-PS Converter  PhysicalDomain=network_engine_domain  SubClassName=ps_input  LeftPortType=input  RightPortType=output  PseudoPeriodic=off  Frequencies=[]  NoiseDistribution=none  NoiseParameters=[]  Unit=kg/s  AffineConversion=off  FilteringAndDerivatives=provide  SimscapeFilterOrder=1  InputFilterTimeConstant=0.001  UdotUserProvided=0
      settings: SourceProductBaseCode=SS,PW,VE
  Simulink-PS Converter2 : nesl_utility/Simulink-PS Converter  PhysicalDomain=network_engine_domain  SubClassName=ps_input  LeftPortType=input  RightPortType=output  PseudoPeriodic=off  Frequencies=[]  NoiseDistribution=none  NoiseParameters=[]  Unit=kg/s  AffineConversion=off  FilteringAndDerivatives=provide  SimscapeFilterOrder=1  InputFilterTimeConstant=0.001  UdotUserProvided=0
      settings: SourceProductBaseCode=SS,PW,VE
  Subtract : Sum  Inputs=-+
  Subtract1 : Sum  Inputs=+-
  Subtract2 : Sum  Inputs=-+
  Switch{,1..3} (4 alike) : Switch  Threshold=1  SaturateOnIntegerOverflow=off  InputSameDT=off
  Switch4 : Switch  Criteria=u2 > Threshold  Threshold=1  SaturateOnIntegerOverflow=off  InputSameDT=off
  Upstream Pres : nesl_utility/PS-Simulink Converter  PhysicalDomain=network_engine_domain  SubClassName=ps_output  LeftPortType=input  RightPortType=output  PseudoPeriodic=off  Frequencies=[]  VectorFormat=1-D array  Unit=inherit  AffineConversion=off
      settings: SourceProductBaseCode=SS,PW,VE
  Upstream Pres1 : nesl_utility/PS-Simulink Converter  PhysicalDomain=network_engine_domain  SubClassName=ps_output  LeftPortType=input  RightPortType=output  PseudoPeriodic=off  Frequencies=[]  VectorFormat=1-D array  Unit=inherit  AffineConversion=off
      settings: SourceProductBaseCode=SS,PW,VE
  Upstream Pres2 : nesl_utility/PS-Simulink Converter  PhysicalDomain=network_engine_domain  SubClassName=ps_output  LeftPortType=input  RightPortType=output  PseudoPeriodic=off  Frequencies=[]  VectorFormat=1-D array  Unit=inherit  AffineConversion=off
      settings: SourceProductBaseCode=SS,PW,VE
  element : Constant  Value=9
  kg/mol : Constant  Value=0.04401
  kg/mol1 : Constant  Value=0
  kg/mol2 : Constant  Value=8e-9
  kn1 : Gain  Gain=0.37
  q_star1 : MATLAB Function  TreatAsAtomicUnit=on
  spatial_calc1 : MATLAB Function  TreatAsAtomicUnit=on
  T : PMIOPort  Side=Left
  Bed in Temp : PMIOPort  Port=2  Side=Right
  Ads_CO2 : PMIOPort  Port=3  Side=Right
  CO2 on/off : PMIOPort  Port=4  Side=Right
  y : Outport
  wires:
  Product/1 -> Product1/2
  element/1 -> Index Vector/1
  kg/mol/1 -> Product/1
  V/1 -> Product1/1, Constants1/3(V)
  Index Vector/1 -> CO2 plot/1, Product/2  "mol/m3"
  Upstream Pres/1 -> q_star1/2(T), spatial_calc1/4(T)
  Integrator4/1 -> spatial_calc1/2(c), Scope2/1, Index Vector/2, q_star1/1(c_t)  "c/t"
  Constants1/6(cFeed) -> Scope2/2
  Bed length/1 -> spatial_calc1/1(L)
  Constants1/7(delta_eps) -> Roh (kg/m3)/1  "dq/dt"
  Constants1/3(DL) -> spatial_calc1/8(DL), Product3/2
  Constants1/1(eps) -> spatial_calc1/6(eps)
  spatial_calc1/1(D2cDz2) -> Product3/1
  Roh (kg/m3)/1 -> Product5/1  "dq/dt"
  Subtract1/1 -> kn1/1
  Product3/1 -> Add1/1
  Constants1/5(c_init) -> Integrator4/3
  Integrator3/1 -> Subtract1/2, Scope3/1  "q"
  Product4/1 -> Add1/2
  Product5/1 -> Add1/3
  Constants1/2(vs) -> spatial_calc1/7(Vs)
  spatial_calc1/2(DcDz) -> Product4/1
  q_star1/1(q_star) -> Subtract1/1
  Switch3/1 -> Constants1/6(P), spatial_calc1/5(P)
  Constants1/4(vi) -> Product4/2
  Upstream Pres1/1 -> Switch1/2, Integrator3/2, Switch3/2, Switch/2, Integrator4/2, Switch2/2
  Switch/1 -> Constants1/4(CO2), spatial_calc1/3(CO2)
  Mol/1 -> Switch/3
  kn1/1 -> Switch1/1  "dq/dt"
  Switch1/1 -> Product5/2, Integrator3/1
  Mol1/1 -> Switch1/3
  Add1/1 -> Switch2/1
  Switch2/1 -> Integrator4/1
  Const/1 -> Switch2/3
  Constants1/8(q_init) -> Integrator3/3
  resid_CO2/1 -> Constants1/2(resid_CO2)
  Clock/1 -> Constants1/1(time)
  Saturation/1 -> Switch/1
  CO2_mol/mol/1 -> Saturation/1
  Product1/1 -> Simulink-PS Converter1/1, Subtract/2
  P/1 -> Switch3/1
  Mol2/1 -> Switch3/3
  Upstream Pres2/1 -> Constants1/5(T)
  CO2_in_kg/s/1 -> Subtract2/1, Subtract/1
  Switch4/1 -> Simulink-PS Converter/1, y/1, Remv CO2/1
  cycle_time/1 -> Switch4/2
  Subtract/1 -> Switch4/1
  kg/mol1/1 -> Switch4/3
  Subtract2/1 -> Simulink-PS Converter2/1
  kg/mol2/1 -> Subtract2/2
  connections:
  Simulink-PS Converter/RConn1 -- PS Switch/LConn1
  Simulink-PS Converter2/RConn1 -- PS Switch/LConn3
  Upstream Pres/LConn1 -- T/RConn1
  Upstream Pres1/LConn1 -- CO2 on/off/RConn1
  Upstream Pres2/LConn1 -- Bed in Temp/RConn1
  Ads_CO2/RConn1 -- PS Switch/RConn1
  Simulink-PS Converter1/RConn1 -- PS Switch/LConn2

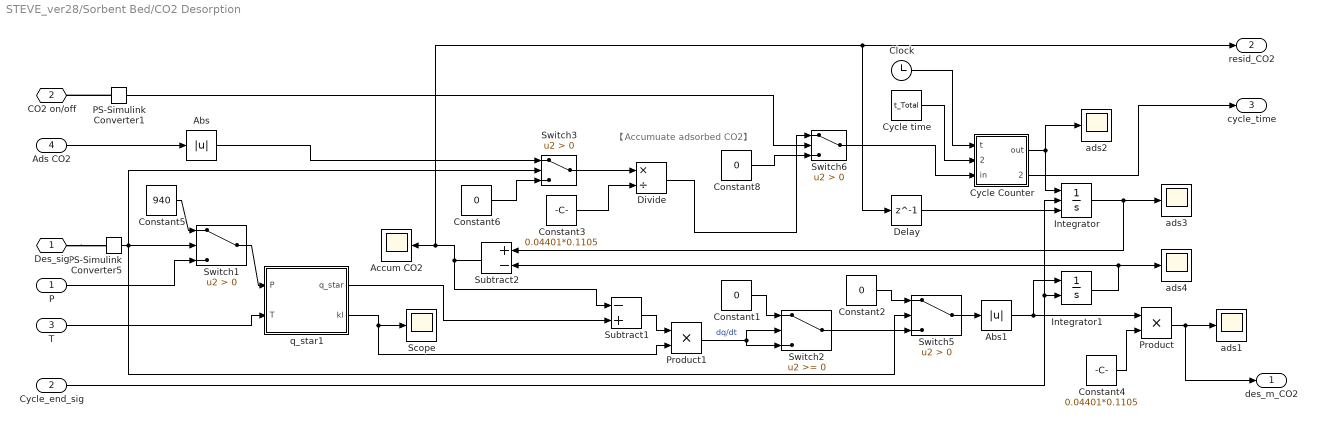
== system STEVE_ver28/Sorbent Bed/CO2 Desorption ==
  note: 【Accumuate adsorbed CO2】
  P : Inport
  Cycle_end_sig : Inport  Port=2
  T : Inport  Port=3
  Ads CO2 : Inport  Port=4
  Abs : Abs  SaturateOnIntegerOverflow=off
  Abs1 : Abs  SaturateOnIntegerOverflow=off
  Accum CO2 : Scope
  Clock : Clock
  Constant{1..2,6,8} (4 alike) : Constant  Value=0
  Constant3 : Constant  Value=0.04401*0.1105
  Constant4 : Constant  Value=0.04401*0.1105
  Constant5 : Constant  Value=940
  Cycle Counter : MATLAB Function  TreatAsAtomicUnit=on
  Cycle time : Constant  Value=t_Total
  Delay : Delay  DelayLength=1  InitialCondition=0
  Divide : Product  Inputs=*/
  Integrator : Integrator  ExternalReset=either  InitialConditionSource=external
  Integrator1 : Integrator  ExternalReset=either
  PS-Simulink Converter1 : nesl_utility/PS-Simulink Converter  PhysicalDomain=network_engine_domain  SubClassName=ps_output  LeftPortType=input  RightPortType=output  PseudoPeriodic=off  Frequencies=[]  VectorFormat=1-D array  Unit=inherit  AffineConversion=off
      settings: SourceProductBaseCode=SS,PW,VE
  PS-Simulink Converter5 : nesl_utility/PS-Simulink Converter  PhysicalDomain=network_engine_domain  SubClassName=ps_output  LeftPortType=input  RightPortType=output  PseudoPeriodic=off  Frequencies=[]  VectorFormat=1-D array  Unit=inherit  AffineConversion=off
      settings: SourceProductBaseCode=SS,PW,VE
  Product : Product
  Product1 : Product
  Scope : Scope
  Subtract1 : Sum  Inputs=-+
  Subtract2 : Sum  Inputs=+-
  Switch{1,3,5..6} (4 alike) : Switch  Criteria=u2 > Threshold  SaturateOnIntegerOverflow=off  InputSameDT=off
  Switch2 : Switch  SaturateOnIntegerOverflow=off  InputSameDT=off
  ads{1..4} (4 alike) : Scope
  q_star1 : MATLAB Function  TreatAsAtomicUnit=on
  Des_sig : PMIOPort  Side=Left
  CO2 on/off : PMIOPort  Port=2  Side=Left
  des_m_CO2 : Outport
  resid_CO2 : Outport  Port=2
  cycle_time : Outport  Port=3
  wires:
  Ads CO2/1 -> Abs/1
  T/1 -> q_star1/2(T)
  Subtract1/1 -> Product1/1
  Product1/1 -> Switch2/2, Switch2/3  "dq/dt"
  Constant1/1 -> Switch2/1
  Constant3/1 -> Divide/2
  Constant4/1 -> Product/2
  Switch1/1 -> q_star1/1(P)
  PS-Simulink Converter5/1 -> Switch1/2, Switch5/2, Switch3/2
  P/1 -> Switch1/3
  Constant5/1 -> Switch1/1
  Abs/1 -> Switch3/1
  Constant6/1 -> Switch3/3
  Switch3/1 -> Divide/1
  Integrator/1 -> ads3/1, Subtract2/1
  Constant2/1 -> Switch5/1
  PS-Simulink Converter1/1 -> Switch6/2
  Divide/1 -> Switch6/1
  Constant8/1 -> Switch6/3
  Product/1 -> des_m_CO2/1, ads1/1
  Switch2/1 -> Switch5/3
  Subtract2/1 -> Subtract1/1, Delay/1, resid_CO2/1, Accum CO2/1
  Integrator1/1 -> Subtract2/2, ads4/1
  Cycle_end_sig/1 -> Integrator1/2, Integrator/2
  Switch5/1 -> Abs1/1
  Abs1/1 -> Integrator1/1, Product/1
  Clock/1 -> Cycle Counter/1(t)
  Cycle time/1 -> Cycle Counter/2(t_tot)
  Switch6/1 -> Cycle Counter/3(in)
  Cycle Counter/1(out) -> Integrator/1, ads2/1
  q_star1/2(kl) -> Scope/1, Product1/2
  q_star1/1(q_star) -> Subtract1/2
  Cycle Counter/2(time) -> cycle_time/1
  Delay/1 -> Integrator/3
  connections:
  Des_sig/RConn1 -- PS-Simulink Converter5/LConn1
  PS-Simulink Converter1/LConn1 -- CO2 on/off/RConn1
